simulink model "controllo_test"  (R2020a)
settings: Solver=VariableStepAuto  StartTime=0.0  StopTime=100  RelTol=1e-3
values from neighbouring files (symbols this model uses):
  a = 0.35    [data.m]    (also in geodetic2nedS.m = 6378137)
  a1 = rho * D^4 * alpha1    (= 0.000388302366464)    [data.m]
  a2 = -rho * D^3 * alpha2 * (1 - omega)    (= 0.0037030698432)    [data.m]
  AHRS_bias = [0 0 0]    [data.m]
  AHRS_sample_time = 1/50    (= 0.02)    [data.m]
  AHRS_var = ([1 1 2] * pi/180).^2    [data.m]
  alpha1 = 0.0113    [data.m]
  alpha2 = -0.0091    [data.m]
  c = son2(1)    [Sonar_id.m]    (also in data.m = 0.19)
  current = [seaCurrent; 0; 0; 0]    [data.m]
  D = 0.076    [data.m]
  dead_zone_limit = 31.5    [data.m]
  DVL_sample_t = 1/12    (= 0.0833333333333)    [data.m]
  DVL_var1 = 0.005^2    (= 2.5e-05)    [data.m]
  DVL_var2 = 0.015^2    (= 0.000225)    [data.m]
  DVL_var3 = 0.023^2    (= 0.000529)    [data.m]
  gps_sample_t = 1    [data.m]
  H = eye(3)    [data.m]    (also in navigation_data.m)
  IMU_sample_time = 1/100    (= 0.01)    [data.m]
  initial = []    [data.m]
  INSP = unicode2native(inspectionDirection)    [data.m]
  Ki_bodypos1 = 0    [parametri_PID.m]
  Ki_bodypos2 = 0    [parametri_PID.m]
  Ki_bodypos3 = 0    [parametri_PID.m]
  Ki_bodypos4 = 0    [parametri_PID.m]
  Ki_bodypos5 = 0    [parametri_PID.m]
  Ki_depth1 = 0    [parametri_PID.m]
  Ki_depth2 = 0    [parametri_PID.m]
  Ki_depth3 = 0    [parametri_PID.m]
  Ki_depth4 = 0    [parametri_PID.m]
  Ki_depth5 = 0    [parametri_PID.m]
  Ki_latvel1 = 0    [parametri_PID.m]
  Ki_latvel2 = 0    [parametri_PID.m]
  Ki_latvel3 = 0    [parametri_PID.m]
  Ki_latvel4 = 0    [parametri_PID.m]
  Ki_latvel5 = 0    [parametri_PID.m]
  Ki_P1 = 0    [parametri_PID.m]
  Ki_P2 = 0    [parametri_PID.m]
  Ki_P3 = 0    [parametri_PID.m]
  Ki_P4 = 0    [parametri_PID.m]
  Ki_P5 = 0    [parametri_PID.m]
  Ki_R1 = 0    [parametri_PID.m]
  Ki_R2 = 0    [parametri_PID.m]
  Ki_R3 = 0    [parametri_PID.m]
  Ki_R4 = 0    [parametri_PID.m]
  Ki_R5 = 0    [parametri_PID.m]
  Ki_rel_or1 = 0    [parametri_PID.m]
  Ki_rel_or2 = 0    [parametri_PID.m]
  Ki_rel_or3 = 0    [parametri_PID.m]
  Ki_rel_or4 = 0    [parametri_PID.m]
  Ki_rel_or5 = 0    [parametri_PID.m]
  Ki_reldist1 = 0    [parametri_PID.m]
  Ki_reldist2 = 0    [parametri_PID.m]
  Ki_reldist3 = 0    [parametri_PID.m]
  Ki_reldist4 = 0    [parametri_PID.m]
  Ki_reldist5 = 0    [parametri_PID.m]
  Ki_surge1 = 0    [parametri_PID.m]
  Ki_surge2 = 0    [parametri_PID.m]
  Ki_surge3 = 0    [parametri_PID.m]
  Ki_surge4 = 0    [parametri_PID.m]
  Ki_surge5 = 0    [parametri_PID.m]
  Ki_yaw1 = 0    [parametri_PID.m]
  Ki_yaw2 = 0    [parametri_PID.m]
  Ki_yaw3 = 0    [parametri_PID.m]
  Ki_yaw4 = 0    [parametri_PID.m]
  Ki_yaw5 = 0    [parametri_PID.m]
  Kp_bodypos1 = 0    [parametri_PID.m]
  Kp_bodypos2 = 2    [parametri_PID.m]
  Kp_bodypos3 = 2    [parametri_PID.m]
  Kp_bodypos4 = 2    [parametri_PID.m]
  Kp_bodypos5 = 2    [parametri_PID.m]
  Kp_depth1 = 0    [parametri_PID.m]
  Kp_depth2 = 2    [parametri_PID.m]
  Kp_depth3 = 2    [parametri_PID.m]
  Kp_depth4 = 2    [parametri_PID.m]
  Kp_depth5 = 2    [parametri_PID.m]
  Kp_latvel1 = 0    [parametri_PID.m]
  Kp_latvel2 = 2    [parametri_PID.m]
  Kp_latvel3 = 2    [parametri_PID.m]
  Kp_latvel4 = 2    [parametri_PID.m]
  Kp_latvel5 = 2    [parametri_PID.m]
  Kp_P1 = 0    [parametri_PID.m]
  Kp_P2 = 2    [parametri_PID.m]
  Kp_P3 = 2    [parametri_PID.m]
  Kp_P4 = 2    [parametri_PID.m]
  Kp_P5 = 2    [parametri_PID.m]
  Kp_R1 = 0    [parametri_PID.m]
  Kp_R2 = 2    [parametri_PID.m]
  Kp_R3 = 2    [parametri_PID.m]
  Kp_R4 = 2    [parametri_PID.m]
  Kp_R5 = 2    [parametri_PID.m]
  Kp_rel_or1 = 0    [parametri_PID.m]
  Kp_rel_or2 = 2    [parametri_PID.m]
  Kp_rel_or3 = 2    [parametri_PID.m]
  Kp_rel_or4 = 2    [parametri_PID.m]
  Kp_rel_or5 = 2    [parametri_PID.m]
  Kp_reldist1 = 0    [parametri_PID.m]
  Kp_reldist2 = 2    [parametri_PID.m]
  Kp_reldist3 = 2    [parametri_PID.m]
  Kp_reldist4 = 2    [parametri_PID.m]
  Kp_reldist5 = 2    [parametri_PID.m]
  Kp_surge1 = 0    [parametri_PID.m]
  Kp_surge2 = 2    [parametri_PID.m]
  Kp_surge3 = 2    [parametri_PID.m]
  Kp_surge4 = 2    [parametri_PID.m]
  Kp_surge5 = 2    [parametri_PID.m]
  Kp_yaw1 = 0.6*6    (= 3.6)    [parametri_PID.m]
  Kp_yaw2 = 2    [parametri_PID.m]
  Kp_yaw3 = 2    [parametri_PID.m]
  Kp_yaw4 = 2    [parametri_PID.m]
  Kp_yaw5 = 2    [parametri_PID.m]
  M = M_rb + M_a    [Masse.m]
  M_inv = inv(M)    [Masse.m]
  n_max = 340    [data.m]
  num_cycle = 5    [data.m]    (also in navigation_data.m)
  omega = 0.1    [data.m]
  ps_sample_t = 0.02    [data.m]
  ps_var = (5000/3)^2    (= 2777777.77778)    [data.m]
  pylonCenter = [ 43.723046 ... (first row only)    [missionB.m]
  pylonRadius = 10    [missionB.m]
  ... (+3 more)
undefined symbols (not defined in the file or in its folder): arrival_point, DiscIntNeverNeededParam, Kd_bodypos2, Kd_bodyposy2, Kd_dist_mis2, Kd_surge2, Kd_yaw1, Ki_bodyposy2, Ki_dist_mis2, Kp_dist_mis2, s_data
libraries: simulink x8
(part 1 of 4)
settings Model: Creator=andrea  LastModifiedBy=marco
settings DebuggingCC: ArithmeticOperatorsInVariantConditions=warning
settings SFSimCC: CustomCodeUndefinedFunction=UseInterfaceOnly

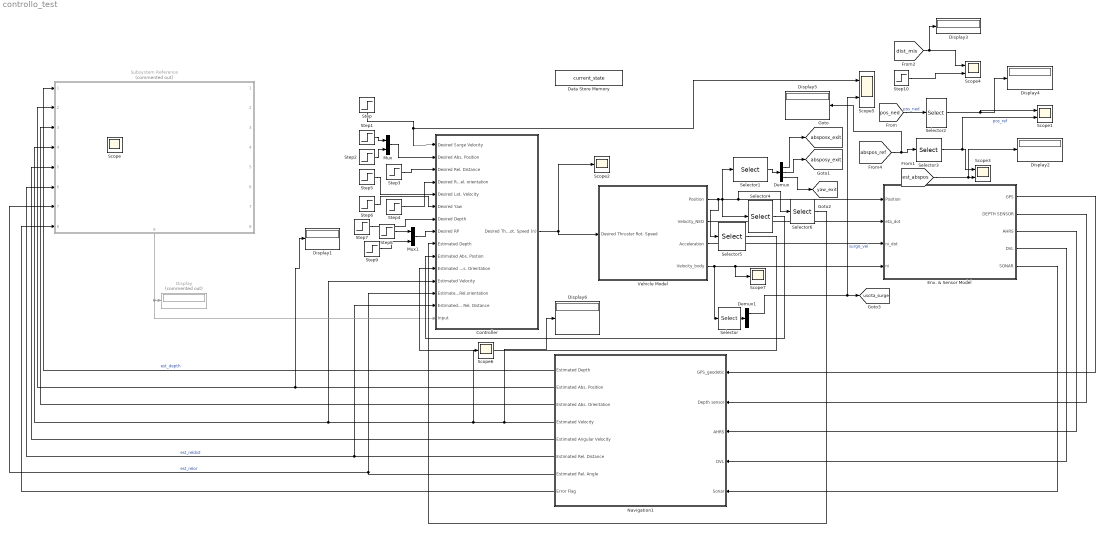
== system controllo_test ==
  Controller : Subsystem
  Data Store Memory : DataStoreMemory  DataStoreName=current_state  ReadBeforeWriteMsg=warning  WriteAfterWriteMsg=warning  WriteAfterReadMsg=warning  ShowAdditionalParam=off
  Demux : Demux  Outputs=3
  Demux1 : Demux  Outputs=2
  Display : Display  Commented=on
  Display{1..6} (6 alike) : Display
  Env. & Sensor Model : Subsystem
  Mux : Mux  Inputs=2
  Mux1 : Mux  Inputs=2
  Navigation1 : Subsystem
  Scope{1,3..5} (4 alike) : Scope  NumInputPorts=2
  Scope{,2,6..7} (4 alike) : Scope
  Selector : Selector  InputPortWidth=6  IndexOptions=Index vector (dialog)  Indices=[1 2 ]  OutputSizes=1
  Selector1 : Selector  InputPortWidth=6  IndexOptions=Index vector (dialog)  Indices=[1 2 6]  OutputSizes=1
  Selector2 : Selector  InputPortWidth=6  IndexOptions=Index vector (dialog)  Indices=[1 2]  OutputSizes=1
  Selector3 : Selector  InputPortWidth=3  IndexOptions=Index vector (dialog)  Indices=[1 2]  OutputSizes=1
  Selector4 : Selector  InputPortWidth=6  IndexOptions=Index vector (dialog)  Indices=[1 2 ]  OutputSizes=1
  Selector5 : Selector  InputPortWidth=6  IndexOptions=Index vector (dialog)  Indices=[4 5 6]  OutputSizes=1
  Selector6 : Selector  InputPortWidth=6  IndexOptions=Index vector (dialog)  Indices=[3]  OutputSizes=1
  Step{,3..8,10} (8 alike) : Step  After=0  SampleTime=0
  Step1 : Step  After=43.722904747658461  SampleTime=0
  Step2 : Step  After=10.396596368122747  SampleTime=0
  Step9 : Step  SampleTime=0
  Subsystem Reference : Subsystem  Commented=on  ReferencedSubsystem=mission_supervisor_sys
      settings: PortSchema="{\"entries\":[{\"content\":{\"sides\":[{\"content\":{\"connectorIds\":[\"In1\",\"In2\",\"In3\",\"In4\",\"In5\",\"In6\",\"In7\",\"In8\"]},\"type\":\"ConnectorPlacement.EquallySpacedRectSide\",\"uuid\":\"88d2dc79-848e-42f0-9e9e-23d8acdf1ba5\"},{\"content\":{\"connectorIds\":[\"Out1\",\"Out2\",\"Out3\",\"Out4\",\"Out5\",\"Out6\",\"Out7\",\"Out8\"],\"side\":\"RIGHT\"},\"type\":\"ConnectorPlacement.EquallySpacedRectSide\",\"uuid\":\"9b84f7d8-cdab-4722-ae5c-2c9e65c7a82f\"},{\"content\":{\"connectorIds\":[],\"side\":\"TOP\"},\"type\":\"ConnectorPlacement.EquallySpacedRectSide\",\"uuid\":\"41854cae-679a-477c-a337-a695a7e6b935\"},{\"content\":{\"connectorIds\":[\"Out9\"],\"side\":\"BOTTOM\"},\"type\":\"ConnectorPlacement.EquallySpacedRectSide\",\"uuid\":\"9cd3ab99-0ab4-4818-acd3-672b60d7f95d\"}]},\"type\":\"ConnectorPlacement.EquallySpacedConnector\",\"uuid\":\"a3d82e32-8d54-4351-960a-48f312f72e96\"}],\"packageUris\":[\"http://schema.mathworks.com/mf0/Connector/19700101\"],\"version\":\"1.0\"}"
  Vehicle Model : Subsystem
      mask Display: image('$imagefile'); % Use "Edit Image" on toolstrip to change.
  tag scope: absposx_exit=global, absposy_exit=global, uscita_surge=global, yaw_exit=global
  wires:
  Controller/1(Desired Thruster Rot. Speed (n)) -> Vehicle Model/1(Desired Thruster Rot. Speed), Scope2/1
  Vehicle Model/1(Position) -> Selector5/1, Selector4/1, Selector1/1, Selector6/1, Env. & Sensor Model/1(Position)
  Env. & Sensor Model/2(DEPTH SENSOR) -> Navigation1/2(Depth sensor)
  Env. & Sensor Model/3(AHRS) -> Navigation1/3(AHRS)
  Navigation1/1(Estimated Depth) -> Subsystem Reference/1  "est_depth"
  Navigation1/3(Estimated Abs. Orientation) -> Subsystem Reference/3
  Navigation1/4(Estimated Velocity) -> Display6/1, Scope6/1, Subsystem Reference/4, Controller/12(Estimated Velocity)
  Vehicle Model/4(Velocity_body) -> Scope7/1, Env. & Sensor Model/4(ni), Selector/1
  Navigation1/6(Estimated Rel. Distance) -> Subsystem Reference/6, Controller/14(Estimated Rel. Distance)  "est_reldist"
  Navigation1/7(Estimated Rel. Angle) -> Subsystem Reference/7, Controller/13(Estimated Rel.orientation)  "est_relor"
  Vehicle Model/2(Velocity_NED) -> Env. & Sensor Model/2(eta_dot)
  Vehicle Model/3(Acceleration) -> Env. & Sensor Model/3(ni_dot)
  Env. & Sensor Model/1(GPS) -> Navigation1/1(GPS_geodetic)
  Env. & Sensor Model/4("DVL ") -> Navigation1/4(DVL)
  Env. & Sensor Model/5(SONAR) -> Navigation1/5(Sonar)
  Subsystem Reference/9 -> Controller/15(Input), Display/1
  Navigation1/5(Estimated Angular Velocity) -> Subsystem Reference/5
  Navigation1/8(Error Flag) -> Subsystem Reference/8
  Step/1 -> Scope5/1, Controller/1(Desired Surge Velocity)
  Step2/1 -> Mux/2
  Mux/1 -> Controller/2(Desired Abs. Position)
  Selector/1 -> Demux1/1
  Demux1/1 -> Scope5/2, [uscita_surge]  "surge_vel"
  Step3/1 -> Controller/3(Desired Rel. Distance)
  Step4/1 -> Controller/4(Desired Rel. orientation)
  Step5/1 -> Controller/5(Desired Lat. Velocity)
  Step6/1 -> Controller/6(Desired Yaw)
  Step7/1 -> Controller/7(Desired Depth)
  Step9/1 -> Mux1/2
  Step8/1 -> Mux1/1
  Mux1/1 -> Controller/8(Desired RP)
  Step1/1 -> Mux/1
  [abspos_ref] -> Display5/1, Selector3/1
  [pos_ned] -> Selector2/1  "pos_ned"
  Selector3/1 -> Scope1/2, Scope3/1  "pos_ref"
  Selector1/1 -> Demux/1
  Demux/3 -> [yaw_exit]
  Demux/1 -> [absposx_exit]
  Demux/2 -> [absposy_exit]
  [est_abspos] -> Display2/1, Scope3/2
  [dist_mis] -> Display3/1, Scope4/1
  Step10/1 -> Scope4/2
  Selector2/1 -> Scope1/1, Display4/1
  Navigation1/2(Estimated Abs. Position) -> Subsystem Reference/2, Display1/1
  Selector4/1 -> Controller/10(Estimated Abs. Postion)
  Selector5/1 -> Controller/11(Estimated Abs. Orientation)
  Selector6/1 -> Controller/9(Estimated Depth)

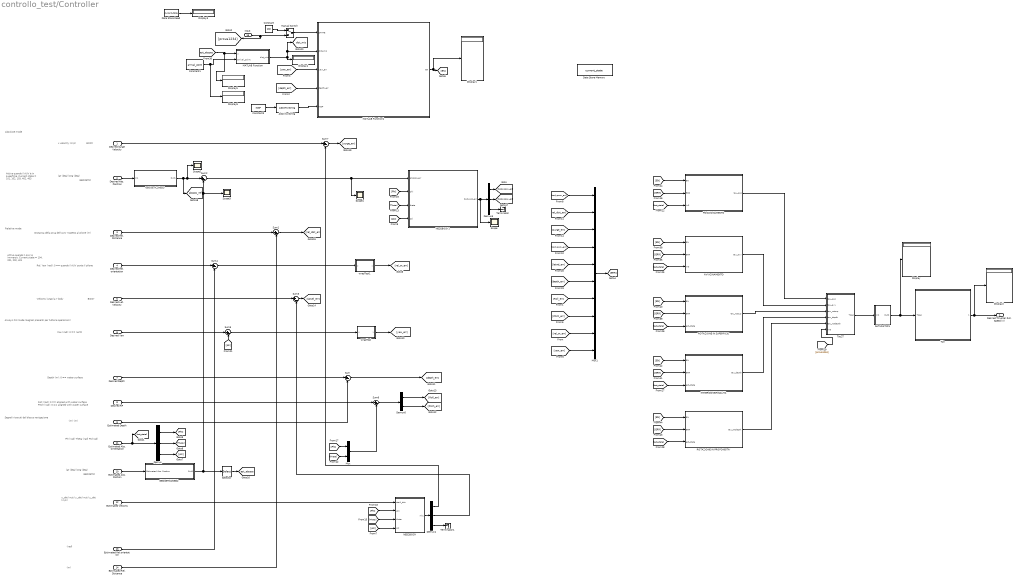
== system controllo_test/Controller ==
  note: lat (deg)
      | long (deg)
  note: (m)
  note: BODY
  note: x velocity (m/s)
  note: lat (deg)
      | long (deg)
  note: GEODETIC
  note: BODY
  note: Relative mode
  note: Absolute mode
  note: GEODETIC
  note: Always ON mode (segnali presenti per tutte le operazioni)
  note: Roll (rad): 0 == aligned with water surface
      | Pitch (rad): 0 == aligned with water surface
  note: Velocity lungo la Y body
  note: Distanza della prua dell'AUV rispetto al pilone (m)
  note: Rel. Yaw (rad): 0 == quando il AUV punta il pilone
  note: Attiva quando il AUV è immerso.
      | Current state = 104, 201, 202, 401
  note: Attiva quando il AUV è in superficie.
      | Current state = 101, 102, 103, 402, 403
  note: Depth (m): 0 == water surface
  note: x_dot        (m/s)
      | y_dot          (m/s)
      | z_dot         (m/s)
  note: (rad)
  note: Segnali ricevuti dal blocco navigazione
  note: (m)
      | (m)
  note: Yaw (rad): 0 == north
  note: Phi (rad)
      | Theta (rad)
      | Psi(rad)
  Desired Surge Velocity : Inport
  Desired Abs. Position : Inport  Port=2  Unit=deg  PortDimensions=2
  Desired Rel. Distance : Inport  Port=3  Unit=m  PortDimensions=1
  Desired Rel. orientation : Inport  Port=4  Unit=rad  PortDimensions=1
  Desired Lat. Velocity : Inport  Port=5  Unit=m/s  PortDimensions=1
  Desired Yaw : Inport  Port=6  Unit=rad  PortDimensions=1
  Desired Depth : Inport  Port=7  Unit=m  PortDimensions=1
  Desired RP : Inport  Port=8  Unit=rad  PortDimensions=2
  Estimated Depth : Inport  Port=9  Unit=m  PortDimensions=1
  Estimated Abs. Postion : Inport  Port=10  Unit=deg  PortDimensions=2
  Estimated Abs. Orientation : Inport  Port=11  Unit=rad  PortDimensions=3
  Estimated Velocity : Inport  Port=12  Unit=m/s  PortDimensions=3
  Estimated Rel.orientation : Inport  Port=13  Unit=rad  PortDimensions=1
  Estimated Rel. Distance : Inport  Port=14  Unit=m  PortDimensions=1
  Input : Inport  Port=15
  ASCII to String : ASCIIToString
  AVVICINAMENTO : Subsystem
  Constant : Constant  Value=102
  Constant1 : Constant  Value=arrival_point
  Constant3 : Constant  Value=INSP  OutDataTypeStr=uint8
  Data Store Memory : DataStoreMemory  DataStoreName=current_state  ReadBeforeWriteMsg=warning  WriteAfterWriteMsg=warning  WriteAfterReadMsg=warning  ShowAdditionalParam=off
  Data Store Read : DataStoreRead  DataStoreName=current_state  SampleTime=0.1
  Demux : Demux  Outputs=3
  Demux1 : Demux  Outputs=3
  Demux5 : Demux  Outputs=3
  Demux6 : Demux  Outputs=2
  Display{,1..6} (7 alike) : Display
  GEODETIC2NED2 : Subsystem
  GEODETIC2NED3 : Subsystem
  IMMERSIONE/RISALITA : Subsystem
  MATLAB Function : MATLAB Function  TreatAsAtomicUnit=on
  MATLAB Function1 : MATLAB Function  TreatAsAtomicUnit=on  SystemSampleTime=0.1
  Manual Switch : ManualSwitch
  Mux : Mux  Inputs=2
  Mux1 : Mux  Inputs=10
  NED2BODY : MATLAB Function  TreatAsAtomicUnit=on
  NED2BODY1 : MATLAB Function  TreatAsAtomicUnit=on
  POSIZIONAMENTO : Subsystem
  ROTAZIONE IN PROFONDITA' : Subsystem
  ROTAZIONE IN SUPERFICIE : Subsystem
  SATURATION : Subsystem
  Scope{,1..3} (4 alike) : Scope
  Selector : Selector  InputPortWidth=3  IndexOptions=Index vector (dialog)  Indices=[1 2]  OutputSizes=1
  Sum{,1..7} (8 alike) : Sum  Inputs=|+-
  T2n : Subsystem
  Tau2T : Subsystem
  Terminator : Terminator
  Terminator1 : Terminator
  wrapTopi : MATLAB Function  TreatAsAtomicUnit=on
  wrapTopi1 : MATLAB Function  TreatAsAtomicUnit=on
  Desired Thruster Rot. Speed (n) : Outport  Unit=rad/s  PortDimensions=7
  tag scope: abspos_ref=global, dist_mis=global, est_abspos=global
  wires:
  Estimated Abs. Orientation/1 -> [est_state], Demux/1
  Desired Depth/1 -> Sum/1
  Estimated Depth/1 -> Sum/2
  Mux/1 -> Sum6/2
  Desired RP/1 -> Sum6/1
  T2n/1(n) -> Display2/1, Desired Thruster Rot. Speed (n)/1
  Desired Lat. Velocity/1 -> Sum3/1
  Desired Rel. Distance/1 -> Sum1/1
  Estimated Rel. Distance/1 -> Sum1/2
  Sum2/1 -> Scope1/1, NED2BODY1/1(abspos_err)
  Desired Abs. Position/1 -> GEODETIC2NED3/1(In1)
  GEODETIC2NED3/1(Out1) -> [abspos_ref], Sum2/1, Scope2/1
  Estimated Abs. Postion/1 -> GEODETIC2NED2/1(Estimated Abs. Postion)
  GEODETIC2NED2/1(Out1) -> Selector/1, Scope3/1, Sum2/2
  Demux1/1 -> Sum7/2
  Demux1/2 -> Sum3/2
  NED2BODY/1(mi1) -> Demux1/1
  Estimated Velocity/1 -> NED2BODY/1(eta1_dot)
  Estimated Rel.orientation/1 -> Sum4/2
  Demux/3 -> [psi]
  [psi] -> NED2BODY/4(psi)
  [psi] -> NED2BODY1/4(psi)
  Demux/2 -> [Theta]
  [Theta] -> Mux/2
  [Theta] -> NED2BODY1/3(theta)
  [Theta] -> NED2BODY/3(theta)
  Demux/1 -> [Phi]
  [Phi] -> Mux/1
  [Phi] -> NED2BODY/2(phi)
  [Phi] -> NED2BODY1/2(phi)
  Tau2T/1(Tdes) -> SATURATION/1(In2)
  SATURATION/1(Out2) -> Display/1, T2n/1(Tdes)
  Desired Rel. orientation/1 -> Sum4/1
  Desired Surge Velocity/1 -> Sum7/1
  [ERR] -> POSIZIONAMENTO/2(ERR)
  [EN] -> POSIZIONAMENTO/1(EN)
  Sum4/1 -> wrapTopi1/1(u)
  Desired Yaw/1 -> Sum5/1
  [psi] -> Sum5/2
  Sum/1 -> [depth_err]
  Sum3/1 -> [latvel_err]
  Sum1/1 -> [rel_dist_err]
  NED2BODY1/1(bodypos_err) -> Scope/1, Demux5/1
  Sum7/1 -> [surge_err]
  Demux5/1 -> [bodyposx_err]
  Demux5/2 -> [bodyposy_err]
  [EN] -> AVVICINAMENTO/1(EN)
  [ERR] -> AVVICINAMENTO/2(ERR)
  [ERR] -> ROTAZIONE IN SUPERFICIE/2(ERR)
  [ERR] -> IMMERSIONE/RISALITA/2(ERR)
  [EN] -> IMMERSIONE/RISALITA/1(EN)
  [ERR] -> ROTAZIONE IN PROFONDITA'/2(ERR)
  [EN] -> ROTAZIONE IN PROFONDITA'/1(EN)
  MATLAB Function1/1(EN) -> [EN], Display1/1
  [bodyposx_err] -> Mux1/1
  [rel_dist_err] -> Mux1/2
  [surge_err] -> Mux1/3
  [bodyposy_err] -> Mux1/4
  [latvel_err] -> Mux1/5
  [depth_err] -> Mux1/6
  Mux1/1 -> [ERR]
  [Roll_err] -> Mux1/7
  [Pitch_err] -> Mux1/8
  [rel_or_err] -> Mux1/9
  [yaw_err] -> Mux1/10
  [EN] -> ROTAZIONE IN SUPERFICIE/1(EN)
  POSIZIONAMENTO/1(tau_pos) -> Tau2T/1(tau_pos)
  AVVICINAMENTO/1(tau_avv) -> Tau2T/2(tau_avv)
  ROTAZIONE IN SUPERFICIE/1(tau_rotsup) -> Tau2T/3(tau_rotsup)
  IMMERSIONE/RISALITA/1(tau_depth) -> Tau2T/4(tau_depth)
  ROTAZIONE IN PROFONDITA'/1(tau_rotdepth) -> Tau2T/5(tau_rotdepth)
  [depth_err] -> MATLAB Function1/4(depth_err)
  [yaw_err] -> MATLAB Function1/3(yaw_err)
  Constant/1 -> Manual Switch/1
  Data Store Read/1 -> Display3/1
  Manual Switch/1 -> MATLAB Function1/1(STATE)
  Demux5/3 -> Terminator/1
  wrapTopi1/1(y) -> [rel_or_err]
  wrapTopi/1(y) -> [yaw_err]
  Sum6/1 -> Demux6/1
  Demux6/1 -> [Roll_err]
  Demux6/2 -> [Pitch_err]
  ASCII to String/1 -> MATLAB Function1/5(INSP)
  Constant3/1 -> ASCII to String/1
  [est_state] -> POSIZIONAMENTO/3(In3)
  [est_state] -> AVVICINAMENTO/3(In3)
  [est_state] -> ROTAZIONE IN SUPERFICIE/3(est_state)
  [est_state] -> IMMERSIONE/RISALITA/3(est_state)
  [est_state] -> ROTAZIONE IN PROFONDITA'/3(est_state)
  Demux1/3 -> Terminator1/1
  Input/1 -> Manual Switch/2, [prova1234]
  [prova1234] -> Tau2T/6(In6)
  Sum5/1 -> wrapTopi/1(u)
  Selector/1 -> [est_abspos]
  [est_abspos] -> Display5/1, MATLAB Function/1(u)
  Constant1/1 -> Display6/1, MATLAB Function/2(arrival_point)
  MATLAB Function/1(dist_mis) -> [dist_mis], MATLAB Function1/2(dist_mis), Display4/1

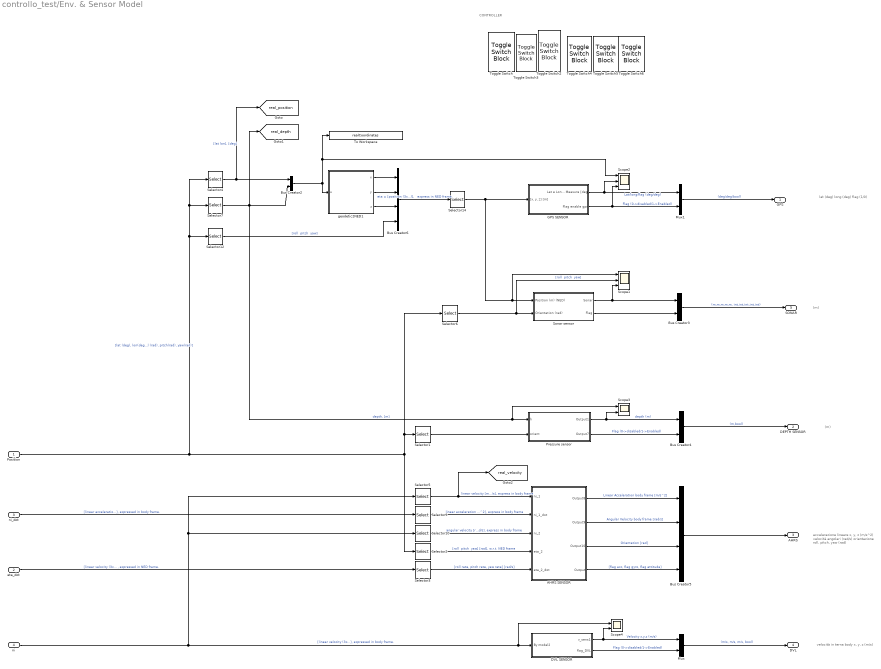
== system controllo_test/Env. & Sensor Model ==
  note: (m)
  note: velocità in terna body x, y, z (m/s)
  note: accelerazione lineare x, y, z (m/s^2)
      | velocità angolari (rad/s)
      | orientazione roll, pitch, yaw (rad)
  note: (m)
  note: lat (deg)
      | long (deg)
      | flag (1/0)
  note: CONTROLLER
  Position : Inport
  eta_dot : Inport  Port=2
  ni_dot : Inport  Port=3
  ni : Inport  Port=4
  AHRS SENSOR : Subsystem
  Bus Creator2 : BusCreator  Inputs=2
  Bus Creator3 : BusCreator  Inputs=2
  Bus Creator4 : BusCreator  Inputs=2
  Bus Creator5 : BusCreator  Inputs=4
  Bus Creator6 : BusCreator  Inputs=4
  DVL SENSOR : Subsystem
  GPS SENSOR : Subsystem
  Mux : Mux  Inputs=2
  Mux1 : Mux  Inputs=2
  Pressure sensor : Subsystem
  Scope1 : Scope  NumInputPorts=3
  Scope2 : Scope  NumInputPorts=3
  Scope3 : Scope  NumInputPorts=2
  Scope4 : Scope  NumInputPorts=2
  Selector{1..3,6,10,12} (6 alike) : Selector  InputPortWidth=6  IndexOptions=Index vector (dialog)  Indices=[4 5 6]  OutputSizes=1
  Selector14 : Selector  InputPortWidth=6  IndexOptions=Index vector (dialog)  Indices=[1 2 3]  OutputSizes=1
  Selector4 : Selector  InputPortWidth=6  IndexOptions=Index vector (dialog)  Indices=[1 2]  OutputSizes=1
  Selector5 : Selector  InputPortWidth=6  IndexOptions=Index vector (dialog)  Indices=[1 2 3]  OutputSizes=1
  Selector7 : Selector  InputPortWidth=6  IndexOptions=Index vector (dialog)  Indices=[3]  OutputSizes=1
  Selector9 : Selector  InputPortWidth=6  IndexOptions=Index vector (dialog)  Indices=[1 2 3]  OutputSizes=1
  Sonar sensor : Subsystem
  To Workspace : ToWorkspace  VariableName=realCoordinates  SampleTime=-1
  Toggle Switch{,2..6} (6 alike) : ToggleSwitchBlock
  geodetic2NED1 : MATLAB Function  TreatAsAtomicUnit=on
  GPS : Outport
  DEPTH SENSOR : Outport  Port=2
  AHRS : Outport  Port=3
  "DVL " : Outport  Port=4
  SONAR : Outport  Port=5
  tag scope: real_depth=global, real_position=global, real_velocity=global
  wires:
  Pressure sensor/1(Output1) -> Bus Creator4/1, Scope3/2  "depth (m)"
  AHRS SENSOR/1(Output8) -> Bus Creator5/1  "Linear Acceleration body frame [m/s^2]"
  Mux1/1 -> GPS/1  "(deg/deg/bool)"
  AHRS SENSOR/3(Output10) -> Bus Creator5/3  "Orientation [rad]"
  Bus Creator6/1 -> Selector14/1  "eta = [position (3x1),  \t  orientation (3x1)], \t  express in NED frame."
  Selector14/1 -> GPS SENSOR/1("[x, y, z] [m]"), Sonar sensor/1(Position (m) (NED)), Scope1/1
  GPS SENSOR/1(Lat e Lon Measure [deg]) -> Scope2/2, Mux1/1  "Lat/long/flag (deg/deg)"
  Selector7/1 -> Bus Creator2/2, [real_depth], Scope3/1, Pressure sensor/1(h)  "depth, [m]"
  geodetic2NED1/3(z) -> Bus Creator6/3
  Selector2/1 -> AHRS SENSOR/4(eta_2)  "[roll  pitch  yaw] [rad], w.r.t. NED frame"
  Bus Creator5/1 -> AHRS/1
  AHRS SENSOR/2(Output9) -> Bus Creator5/2  "Angular Velocity body frame [rad/s]"
  ni/1 -> DVL SENSOR/1(By model2), Scope4/1, Selector10/1, Selector5/1  "[linear velocity (3x1),angular velocity (3x1)], expressed in body frame."
  Selector6/1 -> Sonar sensor/2(Orientation (rad)), Scope1/2  "[roll  pitch  yaw]"
  AHRS SENSOR/4(Output) -> Bus Creator5/4  "[flag acc, flag gyro, flag attitude]"
  GPS SENSOR/2(Flag enable gps) -> Scope2/3, Mux1/2  "Flag (0->disabled/1->Enabled)"
  Selector10/1 -> AHRS SENSOR/3(ni_2)  "angular velocity [rad/s], express in body frame"
  eta_dot/1 -> Selector3/1  "[linear velocity (3x1), roll rate, pitch rate, yaw rate] , expressed in NED frame."
  Selector9/1 -> AHRS SENSOR/2(ni_1_dot)  "linear acceleration [m/s^2], express in body frame"
  Pressure sensor/2(Output7) -> Bus Creator4/2  "Flag (0->disabled/1->Enabled)"
  Selector4/1 -> [real_position], Bus Creator2/1  "[lat lon], [deg]"
  DVL SENSOR/2(flag_DVL) -> Mux/2  "Flag (0->disabled/1->Enabled)"
  Mux/1 -> "DVL "/1  "(m/s, m/s, m/s, bool)"
  geodetic2NED1/1(x) -> Bus Creator6/1
  geodetic2NED1/2(y) -> Bus Creator6/2
  Selector3/1 -> AHRS SENSOR/5(eta_2_dot)  "[roll rate, pitch rate, yaw rate] [rad/s]"
  Sonar sensor/1(Sonar) -> Scope1/3, Bus Creator3/1
  Position/1 -> Selector2/1, Selector1/1, Selector6/1, Selector4/1, Selector7/1, Selector12/1  "[lat (deg), lon(deg), depth(m), roll (rad), pitch(rad), yaw(rad)]"
  Bus Creator4/1 -> DEPTH SENSOR/1  "(m,bool)"
  Selector5/1 -> [real_velocity], AHRS SENSOR/1(ni_1)  "linear velocity [m/s], express in body frame"
  ni_dot/1 -> Selector9/1  "[linear acceleration (3x1), angular acceleration (3x1)], expressed in body frame."
  Bus Creator2/1 -> To Workspace/1, Scope2/1, geodetic2NED1/1(u)
  DVL SENSOR/1(v_sens1) -> Scope4/2, Mux/1  "Velocity x,y,z (m/s)"
  Bus Creator3/1 -> SONAR/1  "(m,m,m,m,m, int,int,int,int,int)"
  Sonar sensor/2(Flag) -> Bus Creator3/2
  Selector12/1 -> Bus Creator6/4  "[roll  pitch  yaw]"
  Selector1/1 -> Pressure sensor/2(orient)

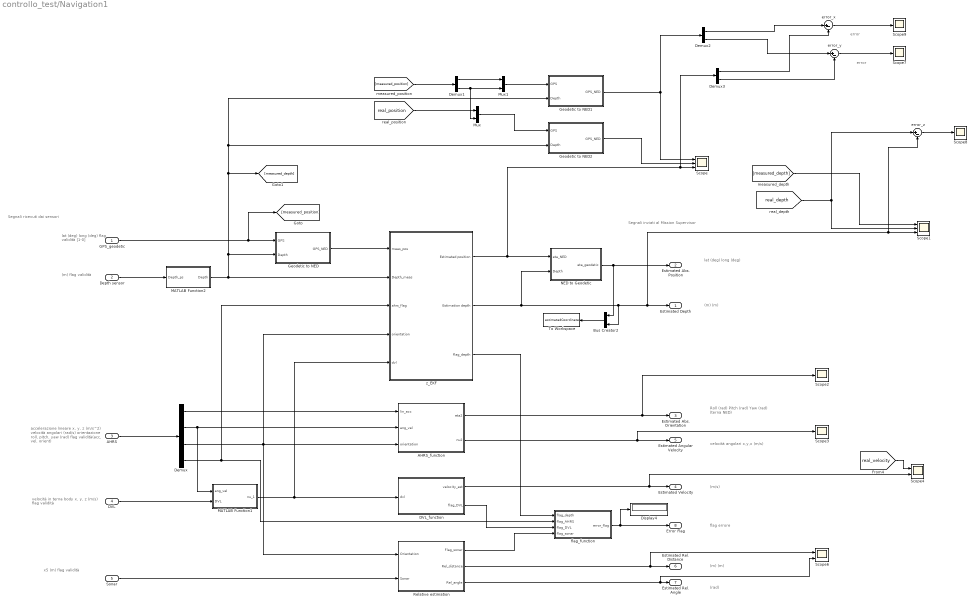
== system controllo_test/Navigation1 ==
  note: (m/s)
  note: (rad)
  note: (m)
      | (m)
  note: (m)
      | flag validità
  note: velocità in terna body x, y, z (m/s)
      | flag validità
  note: error
  note: Segnali ricevuti dai sensori
  note: flag errore
  note: accelerazione lineare x, y, z (m/s^2)
      | velocità angolari (rad/s)
      | orientazione roll, pitch, yaw (rad)
      | flag validità(acc, vel, orient)
  note: velocità angolari x,y,x (m/s)
  note: lat     (deg)
      |  long  (deg)
  note: (m)
      | (m)
  note: Roll (rad)
      | Pitch (rad)
      | Yaw (rad)
      | (terna NED)
  note: x5
      | (m)
      | flag validità
  note: Segnali inviati al Mission Supervisor
  note: error
  note: lat     (deg)
      |  long  (deg)
      | flag validità [1-0]
  GPS_geodetic : Inport  PortDimensions=3
  Depth sensor : Inport  Port=2  PortDimensions=2
  AHRS : Inport  Port=3  PortDimensions=12
  DVL : Inport  Port=4  PortDimensions=4
  Sonar : Inport  Port=5
  AHRS_function : MATLAB Function  TreatAsAtomicUnit=on
  Bus Creator2 : BusCreator  Inputs=2
  DVL_function : MATLAB Function  TreatAsAtomicUnit=on
  Demux : Demux  Outputs=[3 3 3 3]
  Demux1 : Demux  Outputs=2
  Demux2 : Demux  Outputs=2
  Demux3 : Demux  Outputs=2
  Display4 : Display
  Geodetic to NED : Subsystem
  Geodetic to NED1 : Subsystem
  Geodetic to NED2 : Subsystem
  MATLAB Function1 : MATLAB Function  TreatAsAtomicUnit=on  SystemSampleTime=DVL_sample_t
  MATLAB Function2 : MATLAB Function  TreatAsAtomicUnit=on
  Mux : Mux  Inputs=2
  Mux1 : Mux  Inputs=2
  NED to Geodetic : Subsystem
  Relative estimation : Subsystem
  Scope : Scope  NumInputPorts=3
  Scope1 : Scope  NumInputPorts=3
  Scope{2..3,7..9} (5 alike) : Scope
  Scope4 : Scope  NumInputPorts=2
  Scope6 : Scope  NumInputPorts=2
  To Workspace : ToWorkspace  VariableName=estimatedCoordinates  SampleTime=-1
  error_x : Sum  Inputs=|+-
  error_y : Sum  Inputs=|+-
  error_z : Sum  Inputs=|+-
  flag_function : MATLAB Function  TreatAsAtomicUnit=on  SystemSampleTime=1/200
  z_EKF : Subsystem
  Estimated Depth : Outport
  Estimated Abs. Position : Outport  Port=2
  Estimated Abs. Orientation : Outport  Port=3
  Estimated Velocity : Outport  Port=4
  Estimated Angular Velocity : Outport  Port=5
  Estimated Rel. Distance : Outport  Port=6
  Estimated Rel. Angle : Outport  Port=7
  Error Flag : Outport  Port=8
  wires:
  Demux3/1 -> error_x/2
  z_EKF/1(Estimated position) -> Demux3/1, Scope/3, NED to Geodetic/1(eta_NED)
  [real_velocity] -> Scope4/1
  Demux2/2 -> error_y/1
  Relative estimation/1(Flag_sonar) -> flag_function/4(flag_sonar)
  error_x/1 -> Scope9/1
  Mux/1 -> Geodetic to NED2/1(GPS)
  Bus Creator2/1 -> To Workspace/1
  Demux/4 -> z_EKF/3(ahrs_flag), flag_function/2(flag_AHRS)
  MATLAB Function2/1(Depth) -> Geodetic to NED1/2(Depth), Geodetic to NED2/2(Depth), [measured_depth], Geodetic to NED/2(Depth), z_EKF/2(Depth_meas)
  NED to Geodetic/1(eta_geodetic) -> Bus Creator2/1, Estimated Abs. Position/1
  Geodetic to NED1/1(GPS_NED) -> Scope/1, Demux2/1
  z_EKF/3(flag_depth) -> flag_function/1(flag_depth)
  flag_function/1(error_flag) -> Display4/1, Error Flag/1
  AHRS_function/1(eta2) -> Scope2/1, Estimated Abs. Orientation/1
  [real_depth] -> Scope1/2, error_z/1
  Demux3/2 -> error_y/2
  DVL_function/1(velocity_est) -> Scope4/2, Estimated Velocity/1
  AHRS/1 -> Demux/1
  Sonar/1 -> Relative estimation/2(Sonar)
  Demux/2 -> MATLAB Function1/1(ang_vel), AHRS_function/2(ang_vel)
  Demux2/1 -> error_x/1
  Relative estimation/2(Rel_distance) -> Scope6/1, Estimated Rel. Distance/1
  MATLAB Function1/1(nu_1) -> z_EKF/5(dvl), DVL_function/1(dvl)
  Demux1/1 -> Mux1/1
  Demux1/2 -> Mux/2, Mux1/2
  Geodetic to NED/1(GPS_NED) -> z_EKF/1(meas_pos)
  [real_position] -> Mux/1
  error_y/1 -> Scope7/1
  z_EKF/2(Estimation depth) -> NED to Geodetic/2(Depth), Bus Creator2/2, error_z/2, Scope1/3, Estimated Depth/1
  error_z/1 -> Scope8/1
  Relative estimation/3(Rel_angle) -> Scope6/2, Estimated Rel. Angle/1
  [measured_position] -> Demux1/1
  Geodetic to NED2/1(GPS_NED) -> Scope/2
  GPS_geodetic/1 -> Geodetic to NED/1(GPS), [measured_position]
  DVL_function/2(flag_DVL) -> flag_function/3(flag_DVL)
  Depth sensor/1 -> MATLAB Function2/1(Depth_ps)
  Mux1/1 -> Geodetic to NED1/1(GPS)
  DVL/1 -> MATLAB Function1/2(DVL)
  Demux/3 -> z_EKF/4(orientation), AHRS_function/3(orientation), Relative estimation/1(Orientation)
  [measured_depth] -> Scope1/1
  AHRS_function/2(nu2) -> Scope3/1, Estimated Angular Velocity/1
  Demux/1 -> AHRS_function/1(lin_acc)

== system controllo_test/Vehicle Model ==
  note: 3x1 (m/s^2),
      | 3x1 (rad/s^2)
  note: 3x1 (m/s),
      | 3x1 (rad/s)
  note: lat (deg)
      | long (deg)
      | prof. (m),
      | roll (rad),
      | pitch (rad),
      | yaw (rad)
  note: 3x1 (m/s),
      | 3x1 (rad/s)
  Desired Thruster Rot. Speed : Inport
  Add : Sum  Inputs=+-
  Constant : Constant  Value=[100; 100; 0; 0; 0; 0; 0]
  Current : Constant  Value=current
  Demux : Demux
  MATLAB Function : MATLAB Function  TreatAsAtomicUnit=on
  Manual Switch : ManualSwitch  CurrentSetting=0
  Model Vehicle : Subsystem
      mask Display: image('$imagefile'); % Use "Edit Image" on toolstrip to change.
  Scope : Scope
  Scope1 : Scope
  Step : Step  Time=5  Before=[0;0;0;0;0;0;0]  After=[100;-100;0;0;0;0;0]  SampleTime=0
  Thrusters : Subsystem
      mask Display: image('$imagefile'); % Use "Edit Image" on toolstrip to change.
  Position : Outport
  Velocity_NED : Outport  Port=2
  Acceleration : Outport  Port=3
  Velocity_body : Outport  Port=4
  wires:
  Demux/3 -> Velocity_body/1, Add/2  "ni"
  Model Vehicle/1(Out1) -> Demux/1
  Demux/1 -> Thrusters/2(eta), MATLAB Function/1(eta), Position/1, Scope/1  "eta"
  Desired Thruster Rot. Speed/1 -> Manual Switch/2
  Manual Switch/1 -> Thrusters/1(des rot)
  Current/1 -> MATLAB Function/2(current)
  Demux/2 -> Velocity_NED/1  "eta_dot"
  Demux/4 -> Acceleration/1  "ni_dot"
  MATLAB Function/1(ni_c) -> Model Vehicle/2(ni_current), Add/1
  Add/1 -> Thrusters/3(ni)
  Constant/1 -> Manual Switch/1
  Step/1 -> ?
  Thrusters/1(tau) -> Scope1/1, Model Vehicle/1(tau)

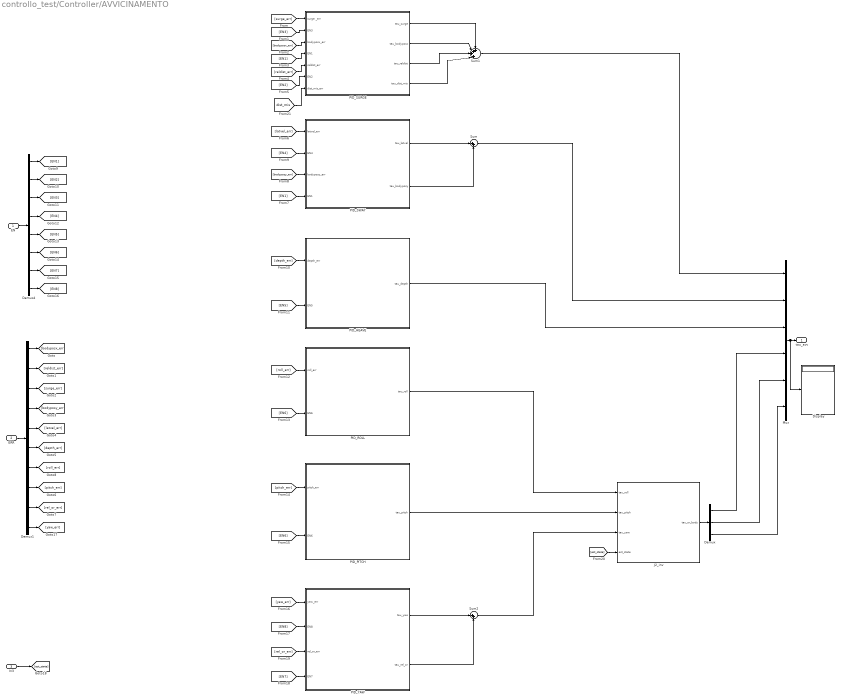
== system controllo_test/Controller/AVVICINAMENTO ==
  EN : Inport
  ERR : Inport  Port=2
  In3 : Inport  Port=3
  Demux : Demux  Outputs=3
  Demux1 : Demux  Outputs=10
  Demux4 : Demux  Outputs=8
  Display : Display
  J2_inv : MATLAB Function  TreatAsAtomicUnit=on
  Mux : Mux  Inputs=6
  PID_HEAVE : Subsystem
  PID_PITCH : Subsystem
  "PID_ROLL " : Subsystem
  PID_SURGE : Subsystem
  PID_SWAY : Subsystem
  PID_YAW : Subsystem
  Sum : Sum  Inputs=|++
  Sum1 : Sum  Inputs=++++|
  Sum2 : Sum  Inputs=|++
  tau_avv : Outport
  wires:
  EN/1 -> Demux4/1
  ERR/1 -> Demux1/1
  Demux4/1 -> [EN1]
  Demux4/2 -> [EN2]
  Demux4/3 -> [EN3]
  Demux4/4 -> [EN4]
  Demux4/5 -> [EN5]
  Demux4/6 -> [EN6]
  Demux4/7 -> [EN7]
  Demux4/8 -> [EN8]
  Demux1/1 -> [bodyposx_err]
  Demux1/2 -> [reldist_err]
  Demux1/3 -> [surge_err]
  Demux1/4 -> [bodyposy_err]
  Demux1/5 -> [latvel_err]
  Demux1/6 -> [depth_err]
  Demux1/7 -> [roll_err]
  Demux1/8 -> [pitch_err]
  Demux1/9 -> [rel_or_err]
  Demux1/10 -> [yaw_err]
  [surge_err] -> PID_SURGE/1(surge _err)
  [EN3] -> PID_SURGE/2(EN3)
  [bodyposx_err] -> PID_SURGE/3(bodyposx_err)
  [EN1] -> PID_SURGE/4(EN1)
  [reldist_err] -> PID_SURGE/5(reldist_err)
  [EN2] -> PID_SURGE/6(EN2)
  [latvel_err] -> PID_SWAY/1(latvel_err)
  [bodyposy_err] -> PID_SWAY/3(bodyposy_err)
  [depth_err] -> PID_HEAVE/1(depth_err)
  [roll_err] -> "PID_ROLL "/1(roll_err)
  [pitch_err] -> PID_PITCH/1(pitch_err)
  [EN6] -> PID_PITCH/2(EN6)
  [yaw_err] -> PID_YAW/1(yaw_err)
  [EN4] -> PID_SWAY/2(EN4)
  [EN1] -> PID_SWAY/4(EN1)
  [EN5] -> PID_HEAVE/2(EN5)
  [EN6] -> "PID_ROLL "/2(EN6)
  [EN8] -> PID_YAW/2("EN8 ")
  [EN7] -> PID_YAW/4(EN7)
  [rel_or_err] -> PID_YAW/3(rel_or_err)
  PID_HEAVE/1(tau_depth) -> Mux/3
  PID_SURGE/1(tau_surge) -> Sum1/1
  Mux/1 -> Display/1, tau_avv/1
  Sum1/1 -> Mux/1
  Sum/1 -> Mux/2
  PID_YAW/1(tau_yaw) -> Sum2/1
  PID_SWAY/2(tau_bodyposy) -> Sum/2
  PID_SURGE/3(tau_reldist) -> Sum1/3
  PID_SURGE/2(tau_bodyposx) -> Sum1/2
  PID_YAW/2(tau_rel_or) -> Sum2/2
  PID_SWAY/1(tau_latvel) -> Sum/1
  Demux/2 -> Mux/5
  PID_PITCH/1(tau_pitch) -> J2_inv/2(tau_pitch)
  J2_inv/1(tau_or_body) -> Demux/1
  Demux/3 -> Mux/6
  "PID_ROLL "/1(tau_roll) -> J2_inv/1(tau_roll)
  Demux/1 -> Mux/4
  [est_state] -> J2_inv/4(est_state)
  Sum2/1 -> J2_inv/3(tau_yaw)
  In3/1 -> [est_state]
  [dist_mis] -> PID_SURGE/7(dist_mis_err)
  PID_SURGE/4(tau_dist_mis) -> Sum1/4

== system controllo_test/Controller/GEODETIC2NED2 ==
  Estimated Abs. Postion : Inport  Unit=deg  PortDimensions=2
  GEODETIC2NED1 : Subsystem
  Out1 : Outport
  wires:
  GEODETIC2NED1/1(Out1) -> Out1/1
  Estimated Abs. Postion/1 -> GEODETIC2NED1/1(In1)

== system controllo_test/Controller/GEODETIC2NED3 ==
  In1 : Inport
  Demux2 : Demux  Outputs=2
  GEODETIC2NED : Subsystem
  Out1 : Outport
  wires:
  Demux2/2 -> GEODETIC2NED/2(lon)
  GEODETIC2NED/1(Out1) -> Out1/1
  Demux2/1 -> GEODETIC2NED/1(lat)
  In1/1 -> Demux2/1

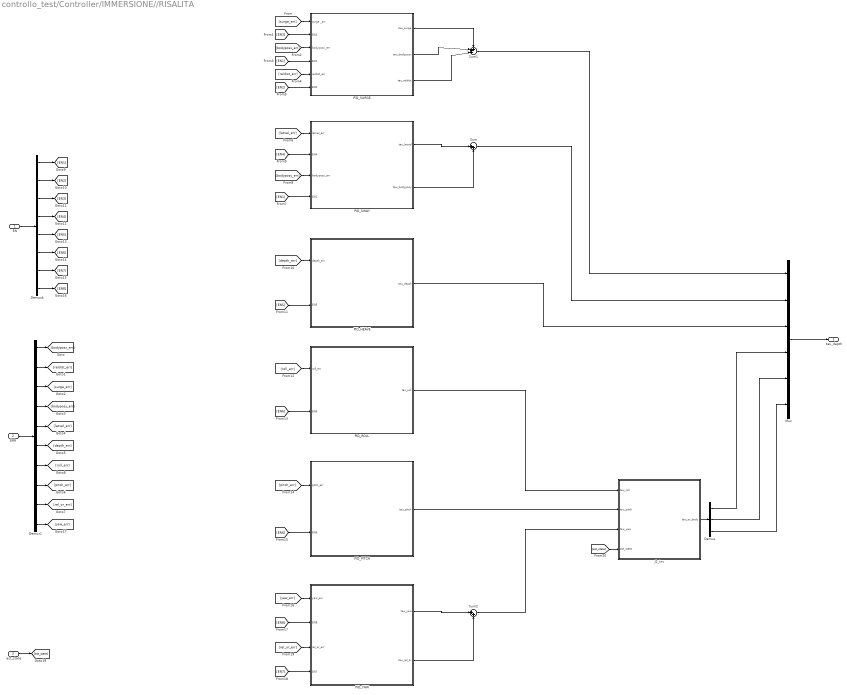
== system controllo_test/Controller/IMMERSIONE//RISALITA ==
  EN : Inport
  ERR : Inport  Port=2
  est_state : Inport  Port=3
  Demux : Demux  Outputs=3
  Demux1 : Demux  Outputs=10
  Demux4 : Demux  Outputs=8
  J2_inv : MATLAB Function  TreatAsAtomicUnit=on
  Mux : Mux  Inputs=6
  PID_HEAVE : Subsystem
  PID_PITCH : Subsystem
  "PID_ROLL " : Subsystem
  PID_SURGE : Subsystem
  PID_SWAY : Subsystem
  PID_YAW : Subsystem
  Sum : Sum  Inputs=|++
  Sum1 : Sum  Inputs=+++|
  Sum2 : Sum  Inputs=|++
  tau_depth : Outport
  wires:
  EN/1 -> Demux4/1
  ERR/1 -> Demux1/1
  Demux4/1 -> [EN1]
  Demux4/2 -> [EN2]
  Demux4/3 -> [EN3]
  Demux4/4 -> [EN4]
  Demux4/5 -> [EN5]
  Demux4/6 -> [EN6]
  Demux4/7 -> [EN7]
  Demux4/8 -> [EN8]
  Demux1/1 -> [bodyposx_err]
  Demux1/2 -> [reldist_err]
  Demux1/3 -> [surge_err]
  Demux1/4 -> [bodyposy_err]
  Demux1/5 -> [latvel_err]
  Demux1/6 -> [depth_err]
  Demux1/7 -> [roll_err]
  Demux1/8 -> [pitch_err]
  Demux1/9 -> [rel_or_err]
  Demux1/10 -> [yaw_err]
  [surge_err] -> PID_SURGE/1(surge _err)
  [EN3] -> PID_SURGE/2(EN3)
  [bodyposx_err] -> PID_SURGE/3(bodyposx_err)
  [EN1] -> PID_SURGE/4(EN1)
  [reldist_err] -> PID_SURGE/5(reldist_err)
  [EN2] -> PID_SURGE/6(EN2)
  [latvel_err] -> PID_SWAY/1(latvel_err)
  [bodyposy_err] -> PID_SWAY/3(bodyposy_err)
  [depth_err] -> PID_HEAVE/1(depth_err)
  [roll_err] -> "PID_ROLL "/1(roll_err)
  [pitch_err] -> PID_PITCH/1(pitch_err)
  [EN6] -> PID_PITCH/2(EN6)
  [yaw_err] -> PID_YAW/1(yaw_err)
  [EN4] -> PID_SWAY/2(EN4)
  [EN1] -> PID_SWAY/4(EN1)
  [EN5] -> PID_HEAVE/2(EN5)
  [EN6] -> "PID_ROLL "/2(EN6)
  [EN8] -> PID_YAW/2("EN8 ")
  [EN7] -> PID_YAW/4(EN7)
  [rel_or_err] -> PID_YAW/3(rel_or_err)
  PID_HEAVE/1(tau_depth) -> Mux/3
  PID_SURGE/1(tau_surge) -> Sum1/1
  Mux/1 -> tau_depth/1
  Sum1/1 -> Mux/1
  Sum/1 -> Mux/2
  PID_YAW/1(tau_yaw) -> Sum2/1
  PID_SWAY/2(tau_bodyposy) -> Sum/2
  PID_SURGE/3(tau_reldist) -> Sum1/3
  PID_SURGE/2(tau_bodyposx) -> Sum1/2
  PID_YAW/2(tau_rel_or) -> Sum2/2
  PID_SWAY/1(tau_latvel) -> Sum/1
  Demux/2 -> Mux/5
  [est_state] -> J2_inv/4(est_state)
  "PID_ROLL "/1(tau_roll) -> J2_inv/1(tau_roll)
  Demux/3 -> Mux/6
  Demux/1 -> Mux/4
  PID_PITCH/1(tau_pitch) -> J2_inv/2(tau_pitch)
  Sum2/1 -> J2_inv/3(tau_yaw)
  J2_inv/1(tau_or_body) -> Demux/1
  est_state/1 -> [est_state]

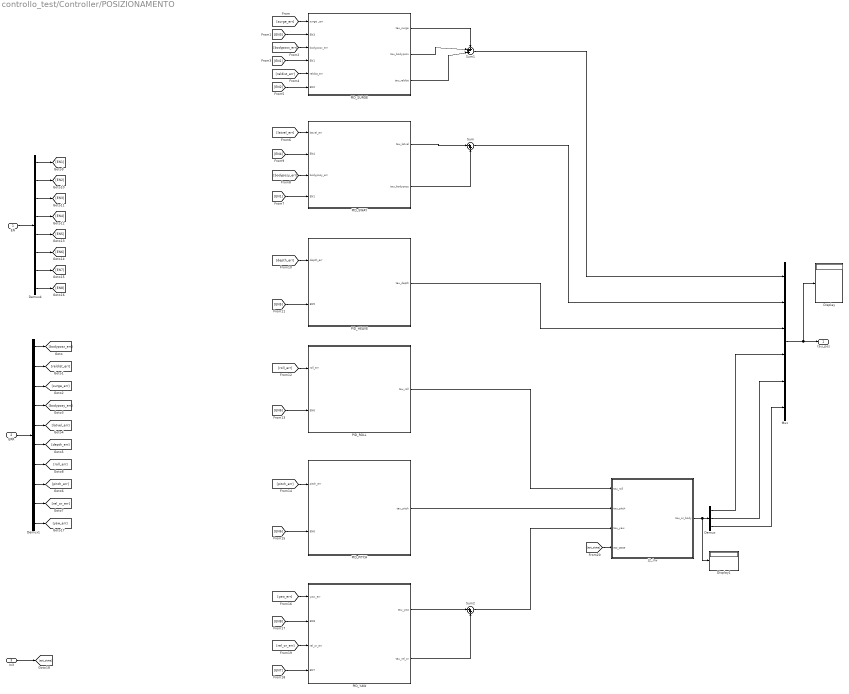
== system controllo_test/Controller/POSIZIONAMENTO ==
  EN : Inport
  ERR : Inport  Port=2
  In3 : Inport  Port=3
  Demux : Demux  Outputs=3
  Demux1 : Demux  Outputs=10
  Demux4 : Demux  Outputs=8
  Display : Display
  Display1 : Display
  J2_inv : MATLAB Function  TreatAsAtomicUnit=on
  Mux : Mux  Inputs=6
  PID_HEAVE : Subsystem
  PID_PITCH : Subsystem
  "PID_ROLL " : Subsystem
  PID_SURGE : Subsystem
  PID_SWAY : Subsystem
  PID_YAW : Subsystem
  Sum : Sum  Inputs=|++
  Sum1 : Sum  Inputs=+++|
  Sum2 : Sum  Inputs=|++
  tau_pos : Outport
  wires:
  PID_SWAY/1(tau_latvel) -> Sum/1
  PID_YAW/2(tau_rel_or) -> Sum2/2
  PID_SURGE/2(tau_bodyposx) -> Sum1/2
  PID_SURGE/3(tau_reldist) -> Sum1/3
  PID_SWAY/2(tau_bodyposy) -> Sum/2
  PID_YAW/1(tau_yaw) -> Sum2/1
  Sum/1 -> Mux/2
  Sum1/1 -> Mux/1
  Mux/1 -> Display/1, tau_pos/1
  PID_SURGE/1(tau_surge) -> Sum1/1
  PID_HEAVE/1(tau_depth) -> Mux/3
  [rel_or_err] -> PID_YAW/3(rel_or_err)
  [EN7] -> PID_YAW/4(EN7)
  [EN8] -> PID_YAW/2("EN8 ")
  [EN6] -> "PID_ROLL "/2(EN6)
  [EN5] -> PID_HEAVE/2(EN5)
  [EN1] -> PID_SWAY/4(EN1)
  [EN4] -> PID_SWAY/2(EN4)
  [yaw_err] -> PID_YAW/1(yaw_err)
  [EN6] -> PID_PITCH/2(EN6)
  [pitch_err] -> PID_PITCH/1(pitch_err)
  [roll_err] -> "PID_ROLL "/1(roll_err)
  [depth_err] -> PID_HEAVE/1(depth_err)
  [bodyposy_err] -> PID_SWAY/3(bodyposy_err)
  [latvel_err] -> PID_SWAY/1(latvel_err)
  [EN2] -> PID_SURGE/6(EN2)
  [reldist_err] -> PID_SURGE/5(reldist_err)
  [EN1] -> PID_SURGE/4(EN1)
  [bodyposx_err] -> PID_SURGE/3(bodyposx_err)
  [EN3] -> PID_SURGE/2(EN3)
  [surge_err] -> PID_SURGE/1(surge _err)
  Demux1/10 -> [yaw_err]
  Demux1/9 -> [rel_or_err]
  Demux1/8 -> [pitch_err]
  Demux1/7 -> [roll_err]
  Demux1/6 -> [depth_err]
  Demux1/5 -> [latvel_err]
  Demux1/4 -> [bodyposy_err]
  Demux1/3 -> [surge_err]
  Demux1/2 -> [reldist_err]
  Demux1/1 -> [bodyposx_err]
  Demux4/8 -> [EN8]
  Demux4/7 -> [EN7]
  Demux4/6 -> [EN6]
  Demux4/5 -> [EN5]
  Demux4/4 -> [EN4]
  Demux4/3 -> [EN3]
  Demux4/2 -> [EN2]
  Demux4/1 -> [EN1]
  ERR/1 -> Demux1/1
  EN/1 -> Demux4/1
  In3/1 -> [est_state]
  [est_state] -> J2_inv/4(est_state)
  "PID_ROLL "/1(tau_roll) -> J2_inv/1(tau_roll)
  PID_PITCH/1(tau_pitch) -> J2_inv/2(tau_pitch)
  Sum2/1 -> J2_inv/3(tau_yaw)
  J2_inv/1(tau_or_body) -> Display1/1, Demux/1
  Demux/1 -> Mux/4
  Demux/2 -> Mux/5
  Demux/3 -> Mux/6

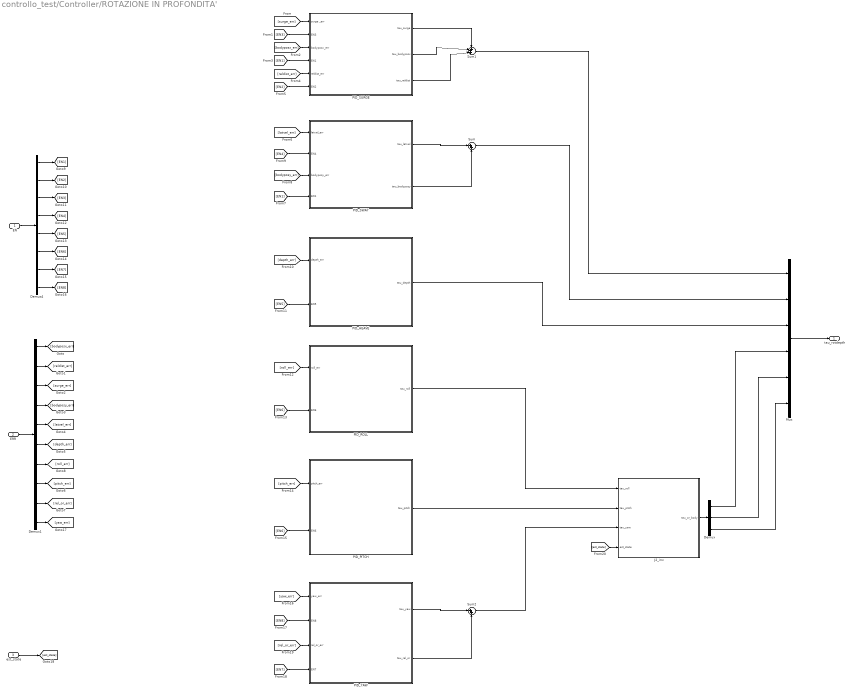
== system controllo_test/Controller/ROTAZIONE IN PROFONDITA' ==
  EN : Inport
  ERR : Inport  Port=2
  est_state : Inport  Port=3
  Demux : Demux  Outputs=3
  Demux1 : Demux  Outputs=10
  Demux4 : Demux  Outputs=8
  J2_inv : MATLAB Function  TreatAsAtomicUnit=on
  Mux : Mux  Inputs=6
  PID_HEAVE : Subsystem
  PID_PITCH : Subsystem
  "PID_ROLL " : Subsystem
  PID_SURGE : Subsystem
  PID_SWAY : Subsystem
  PID_YAW : Subsystem
  Sum : Sum  Inputs=|++
  Sum1 : Sum  Inputs=+++|
  Sum2 : Sum  Inputs=|++
  tau_rotdepth : Outport
  wires:
  EN/1 -> Demux4/1
  ERR/1 -> Demux1/1
  Demux4/1 -> [EN1]
  Demux4/2 -> [EN2]
  Demux4/3 -> [EN3]
  Demux4/4 -> [EN4]
  Demux4/5 -> [EN5]
  Demux4/6 -> [EN6]
  Demux4/7 -> [EN7]
  Demux4/8 -> [EN8]
  Demux1/1 -> [bodyposx_err]
  Demux1/2 -> [reldist_err]
  Demux1/3 -> [surge_err]
  Demux1/4 -> [bodyposy_err]
  Demux1/5 -> [latvel_err]
  Demux1/6 -> [depth_err]
  Demux1/7 -> [roll_err]
  Demux1/8 -> [pitch_err]
  Demux1/9 -> [rel_or_err]
  Demux1/10 -> [yaw_err]
  [surge_err] -> PID_SURGE/1(surge _err)
  [EN3] -> PID_SURGE/2(EN3)
  [bodyposx_err] -> PID_SURGE/3(bodyposx_err)
  [EN1] -> PID_SURGE/4(EN1)
  [reldist_err] -> PID_SURGE/5(reldist_err)
  [EN2] -> PID_SURGE/6(EN2)
  [latvel_err] -> PID_SWAY/1(latvel_err)
  [bodyposy_err] -> PID_SWAY/3(bodyposy_err)
  [depth_err] -> PID_HEAVE/1(depth_err)
  [roll_err] -> "PID_ROLL "/1(roll_err)
  [pitch_err] -> PID_PITCH/1(pitch_err)
  [EN6] -> PID_PITCH/2(EN6)
  [yaw_err] -> PID_YAW/1(yaw_err)
  [EN4] -> PID_SWAY/2(EN4)
  [EN1] -> PID_SWAY/4(EN1)
  [EN5] -> PID_HEAVE/2(EN5)
  [EN6] -> "PID_ROLL "/2(EN6)
  [EN8] -> PID_YAW/2("EN8 ")
  [EN7] -> PID_YAW/4(EN7)
  [rel_or_err] -> PID_YAW/3(rel_or_err)
  PID_HEAVE/1(tau_depth) -> Mux/3
  PID_SURGE/1(tau_surge) -> Sum1/1
  Mux/1 -> tau_rotdepth/1
  Sum1/1 -> Mux/1
  Sum/1 -> Mux/2
  PID_YAW/1(tau_yaw) -> Sum2/1
  PID_SWAY/2(tau_bodyposy) -> Sum/2
  PID_SURGE/3(tau_reldist) -> Sum1/3
  PID_SURGE/2(tau_bodyposx) -> Sum1/2
  PID_YAW/2(tau_rel_or) -> Sum2/2
  PID_SWAY/1(tau_latvel) -> Sum/1
  Demux/1 -> Mux/4
  Sum2/1 -> J2_inv/3(tau_yaw)
  Demux/3 -> Mux/6
  "PID_ROLL "/1(tau_roll) -> J2_inv/1(tau_roll)
  Demux/2 -> Mux/5
  [est_state] -> J2_inv/4(est_state)
  PID_PITCH/1(tau_pitch) -> J2_inv/2(tau_pitch)
  J2_inv/1(tau_or_body) -> Demux/1
  est_state/1 -> [est_state]

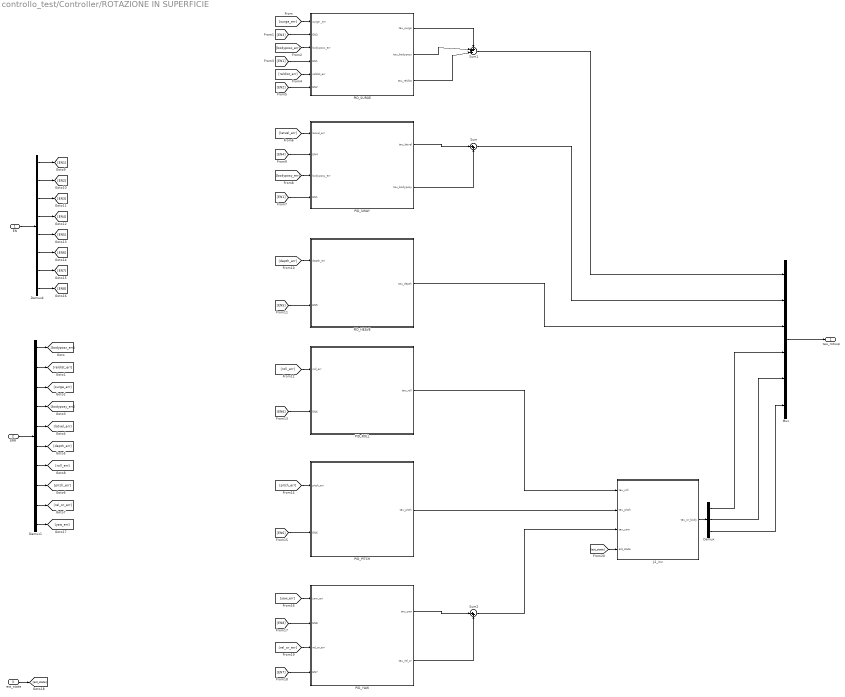
== system controllo_test/Controller/ROTAZIONE IN SUPERFICIE ==
  EN : Inport
  ERR : Inport  Port=2
  est_state : Inport  Port=3
  Demux : Demux  Outputs=3
  Demux1 : Demux  Outputs=10
  Demux4 : Demux  Outputs=8
  J2_inv : MATLAB Function  TreatAsAtomicUnit=on
  Mux : Mux  Inputs=6
  PID_HEAVE : Subsystem
  PID_PITCH : Subsystem
  "PID_ROLL " : Subsystem
  PID_SURGE : Subsystem
  PID_SWAY : Subsystem
  PID_YAW : Subsystem
  Sum : Sum  Inputs=|++
  Sum1 : Sum  Inputs=+++|
  Sum2 : Sum  Inputs=|++
  tau_rotsup : Outport
  wires:
  EN/1 -> Demux4/1
  ERR/1 -> Demux1/1
  Demux4/1 -> [EN1]
  Demux4/2 -> [EN2]
  Demux4/3 -> [EN3]
  Demux4/4 -> [EN4]
  Demux4/5 -> [EN5]
  Demux4/6 -> [EN6]
  Demux4/7 -> [EN7]
  Demux4/8 -> [EN8]
  Demux1/1 -> [bodyposx_err]
  Demux1/2 -> [reldist_err]
  Demux1/3 -> [surge_err]
  Demux1/4 -> [bodyposy_err]
  Demux1/5 -> [latvel_err]
  Demux1/6 -> [depth_err]
  Demux1/7 -> [roll_err]
  Demux1/8 -> [pitch_err]
  Demux1/9 -> [rel_or_err]
  Demux1/10 -> [yaw_err]
  [surge_err] -> PID_SURGE/1(surge _err)
  [EN3] -> PID_SURGE/2(EN3)
  [bodyposx_err] -> PID_SURGE/3(bodyposx_err)
  [EN1] -> PID_SURGE/4(EN1)
  [reldist_err] -> PID_SURGE/5(reldist_err)
  [EN2] -> PID_SURGE/6(EN2)
  [latvel_err] -> PID_SWAY/1(latvel_err)
  [bodyposy_err] -> PID_SWAY/3(bodyposy_err)
  [depth_err] -> PID_HEAVE/1(depth_err)
  [roll_err] -> "PID_ROLL "/1(roll_err)
  [pitch_err] -> PID_PITCH/1(pitch_err)
  [EN6] -> PID_PITCH/2(EN6)
  [yaw_err] -> PID_YAW/1(yaw_err)
  [EN4] -> PID_SWAY/2(EN4)
  [EN1] -> PID_SWAY/4(EN1)
  [EN5] -> PID_HEAVE/2(EN5)
  [EN6] -> "PID_ROLL "/2(EN6)
  [EN8] -> PID_YAW/2("EN8 ")
  [EN7] -> PID_YAW/4(EN7)
  [rel_or_err] -> PID_YAW/3(rel_or_err)
  PID_HEAVE/1(tau_depth) -> Mux/3
  PID_SURGE/1(tau_surge) -> Sum1/1
  Mux/1 -> tau_rotsup/1
  Sum1/1 -> Mux/1
  Sum/1 -> Mux/2
  PID_YAW/1(tau_yaw) -> Sum2/1
  PID_SWAY/2(tau_bodyposy) -> Sum/2
  PID_SURGE/3(tau_reldist) -> Sum1/3
  PID_SURGE/2(tau_bodyposx) -> Sum1/2
  PID_YAW/2(tau_rel_or) -> Sum2/2
  PID_SWAY/1(tau_latvel) -> Sum/1
  J2_inv/1(tau_or_body) -> Demux/1
  "PID_ROLL "/1(tau_roll) -> J2_inv/1(tau_roll)
  Demux/3 -> Mux/6
  Demux/1 -> Mux/4
  PID_PITCH/1(tau_pitch) -> J2_inv/2(tau_pitch)
  [est_state] -> J2_inv/4(est_state)
  Demux/2 -> Mux/5
  Sum2/1 -> J2_inv/3(tau_yaw)
  est_state/1 -> [est_state]

== system controllo_test/Controller/SATURATION ==
  In2 : Inport
  Saturation3 : Saturate  UpperLimit=45  LowerLimit=-45
  Out2 : Outport
  wires:
  In2/1 -> Saturation3/1
  Saturation3/1 -> Out2/1

== system controllo_test/Controller/T2n ==
  Tdes : Inport
  MATLAB Function : MATLAB Function  TreatAsAtomicUnit=on
  n : Outport  Unit=rad/s  PortDimensions=7
  wires:
  Tdes/1 -> MATLAB Function/1(Tdes)
  MATLAB Function/1(n) -> n/1

== system controllo_test/Controller/Tau2T ==
  tau_pos : Inport
  tau_avv : Inport  Port=2
  tau_rotsup : Inport  Port=3
  tau_depth : Inport  Port=4
  tau_rotdepth : Inport  Port=5
  In6 : Inport  Port=6
  Constant : Constant  Value=102
  Data Store Read : DataStoreRead  DataStoreName=current_state  SampleTime=0.1
  Display : Display
  Display1 : Display
  Manual Switch : ManualSwitch
  Tau2T : MATLAB Function  TreatAsAtomicUnit=on
  Tau_des ENABLE : MATLAB Function  TreatAsAtomicUnit=on
  Tdes : Outport
  wires:
  Tau2T/1(T) -> Display1/1, Tdes/1
  tau_avv/1 -> Tau_des ENABLE/3(tau2)
  tau_rotsup/1 -> Tau_des ENABLE/4(tau3)
  tau_depth/1 -> Tau_des ENABLE/5(tau4)
  tau_rotdepth/1 -> Tau_des ENABLE/6(tau5)
  Tau_des ENABLE/1(tau_des) -> Display/1, Tau2T/1(tau_des)
  Constant/1 -> Manual Switch/1
  Manual Switch/1 -> Tau_des ENABLE/1(STATE)
  In6/1 -> Manual Switch/2
  tau_pos/1 -> Tau_des ENABLE/2(tau1)

== system controllo_test/Env. & Sensor Model/AHRS SENSOR ==
  note: AHRS
      |
      | Dynamic Accuracy (Heading):   2.0° RMS
      | Dynamic Accuracy (Pitch/Roll): 1.0° RMS
  note: Output Rate (IMU Data): 800 Hz
  note: Resolution:
  note: 0.02		      	 °
      | 0.3491 * 10-3 rad
  note: 0.05				°
      | 0,8727 * 10^-3	rad
  note: 0,0015 Gauss
  note: Vectornav VN-100 IMU/AHRS
  note: IMU
  note: 0.05			    mg
      | 0.4905 * 10^-3  m/s^2
  note: Output Rate (Attitude Data): 400 Hz
  ni_1 : Inport  SampleTime=IMU_sample_time
  ni_1_dot : Inport  Port=2  SampleTime=IMU_sample_time
  ni_2 : Inport  Port=3  SampleTime=IMU_sample_time
  eta_2 : Inport  Port=4  SampleTime=AHRS_sample_time
  eta_2_dot : Inport  Port=5  SampleTime=IMU_sample_time
  "   " : MATLAB Function  TreatAsAtomicUnit=on
  ACC : Constant
  AHRS2 : Constant
  Accelerometer : Subsystem
  Bus Creator : BusCreator  Inputs=3
  GYRO : Constant
  Gyroscope : Subsystem
  Magnetometer : Subsystem
  Quantizer : Quantizer  QuantizationInterval=Resolution_acc
  Quantizer1 : Quantizer  QuantizationInterval=Resolution_gyro
  Quantizer2 : Quantizer  QuantizationInterval=Resolution_magn
  Quantizer3 : Quantizer  QuantizationInterval=Resolution_AHRS
  Random Number : RandomNumber  Mean=AHRS_bias  Variance=AHRS_var  Seed=[232 342 202]  SampleTime=AHRS_sample_time
  Scope : Scope
  Sum : Sum  Inputs=|++
  Output8 : Outport  SampleTime=IMU_sample_time
  Output9 : Outport  Port=2  SampleTime=IMU_sample_time
  Output10 : Outport  Port=3  SampleTime=AHRS_sample_time
  Output : Outport  Port=4  SampleTime=AHRS_sample_time
  wires:
  "   "/2(ang_vel) -> Gyroscope/1(In1)
  Gyroscope/1(ang_vel) -> Quantizer1/1
  ni_1/1 -> "   "/1(ni_1)
  eta_2/1 -> Sum/2, "   "/4(eta_2)
  ni_2/1 -> "   "/3(ni_2)
  Quantizer2/1 -> Scope/1
  Quantizer1/1 -> Output9/1
  Accelerometer/1(lin_acc) -> Quantizer/1
  ni_1_dot/1 -> "   "/2(ni_1_dot)
  Sum/1 -> Quantizer3/1
  "   "/1(lin_acc) -> Accelerometer/1(In1)
  Quantizer/1 -> Output8/1
  eta_2_dot/1 -> "   "/5(eta_2_dot)
  Random Number/1 -> Sum/1
  "   "/3(m) -> Magnetometer/1(In1)
  Magnetometer/1(m) -> Quantizer2/1
  Quantizer3/1 -> Output10/1
  ACC/1 -> Bus Creator/1
  GYRO/1 -> Bus Creator/2
  AHRS2/1 -> Bus Creator/3
  Bus Creator/1 -> Output/1

== system controllo_test/Env. & Sensor Model/DVL SENSOR ==
  By model2 : Inport  SampleTime=DVL_sample_t
  AND1 : Logic  IconShape=distinctive  AllPortsSameDT=off  OutDataTypeStr=boolean
  DVL : Constant
  Data Type Conversion : DataTypeConversion  OutDataTypeStr=double
  Demux : Demux  Outputs=3
  MATLAB Function : MATLAB Function  TreatAsAtomicUnit=on
  MATLAB Function2 : MATLAB Function  TreatAsAtomicUnit=on
  Quantizer : Quantizer  QuantizationInterval=DVL_resol
  Selector9 : Selector  InputPortWidth=6  IndexOptions=Index vector (dialog)  Indices=[1 2 3]  OutputSizes=1
  Subsystem : Subsystem
  Subsystem1 : Subsystem
  Subsystem2 : Subsystem
  Sum1 : Sum  Inputs=|++
  Sum2 : Sum  Inputs=|++
  Sum3 : Sum  Inputs=|++
  Vector Concatenate : Concatenate  NumInputs=3
  v_sens1 : Outport  SampleTime=DVL_sample_t
  flag_DVL : Outport  Port=2  SampleTime=DVL_sample_t
  wires:
  MATLAB Function2/1(flag) -> AND1/1
  DVL/1 -> AND1/2
  AND1/1 -> Data Type Conversion/1
  Demux/1 -> Sum1/1, Subsystem/1(In1)
  Subsystem/1(Out1) -> Sum1/2
  Demux/2 -> Sum2/1, Subsystem1/1(In1)
  Subsystem1/1(Out1) -> Sum2/2
  Demux/3 -> Sum3/1, Subsystem2/1(In1)
  Subsystem2/1(Out1) -> Sum3/2
  Sum2/1 -> Vector Concatenate/2
  Sum1/1 -> Vector Concatenate/1
  Sum3/1 -> Vector Concatenate/3
  Vector Concatenate/1 -> Quantizer/1
  By model2/1 -> MATLAB Function/1(ni), Selector9/1
  Quantizer/1 -> v_sens1/1
  Data Type Conversion/1 -> flag_DVL/1
  Selector9/1 -> MATLAB Function2/1(v)
  MATLAB Function/1(niDVL) -> Demux/1

== system controllo_test/Env. & Sensor Model/GPS SENSOR ==
  note: Copernicus II DIP
  note: Control state sensors. 1:enabled, 0:disabled
  "[x, y, z] [m]" : Inport  SampleTime=gps_sample_t
  Add noiose : Subsystem
  Control state : Subsystem
  Demux : Demux  Outputs=3
  NED2Geodetic : MATLAB Function  TreatAsAtomicUnit=on
  Threshold : MATLAB Function  TreatAsAtomicUnit=on
  Zero-Order Hold : ZeroOrderHold  SampleTime=gps_sample_t
  Lat e Lon Measure [deg] : Outport
  Flag enable gps : Outport  Port=2
  wires:
  Threshold/2(x_out) -> Add noiose/1(In1)  "x"
  Threshold/3(y_out) -> Add noiose/2(In2)  "y"
  Threshold/1(depth) -> NED2Geodetic/1(depth)
  Add noiose/1(Out1) -> NED2Geodetic/2(u)  "out"
  Threshold/4(flag_enable_gps) -> Control state/1(In1)
  Control state/1(Flag enable gps) -> NED2Geodetic/3(enableGps), Flag enable gps/1
  NED2Geodetic/1(data_GDT) -> Zero-Order Hold/1
  "[x, y, z] [m]"/1 -> Demux/1
  Demux/1 -> Threshold/1(x_in)
  Demux/2 -> Threshold/2(y_in)
  Demux/3 -> Threshold/3(h_in)
  Zero-Order Hold/1 -> Lat e Lon Measure [deg]/1  "(deg/deg/bool)"

== system controllo_test/Env. & Sensor Model/Pressure sensor ==
  h : Inport  SampleTime=ps_sample_t
  orient : Inport  Port=2
  DEPTH MEASUREMENT : Constant
  MATLAB Function2 : MATLAB Function  TreatAsAtomicUnit=on
  MATLAB Function3 : MATLAB Function  TreatAsAtomicUnit=on
  Quantizer1 : Quantizer  QuantizationInterval=ps_resol  LinearizeAsGain=off
  Random Number1 : RandomNumber  Variance=ps_var  SampleTime=ps_sample_t
  Sum1 : Sum  Inputs=|++
  Zero-Order Hold : ZeroOrderHold  SampleTime=ps_sample_t
  Output1 : Outport  SampleTime=ps_sample_t
  Output7 : Outport  Port=2
  wires:
  DEPTH MEASUREMENT/1 -> Output7/1
  Random Number1/1 -> Sum1/2
  MATLAB Function2/1(p) -> Sum1/1
  MATLAB Function3/1(h) -> Zero-Order Hold/1
  Sum1/1 -> Quantizer1/1
  Quantizer1/1 -> MATLAB Function3/2(p)
  h/1 -> MATLAB Function2/1(h)
  Zero-Order Hold/1 -> Output1/1
  orient/1 -> MATLAB Function3/1(orient)

== system controllo_test/Env. & Sensor Model/Sonar sensor ==
  Position (m) (NED) : Inport  SampleTime=s_data.smpl
  Orientation (rad) : Inport  Port=2  SampleTime=s_data.smpl
  Demux : Demux  Outputs=3
  Demux1 : Demux  Outputs=3
  Gain : Gain  Gain=8*ones(5,1)  Multiplication=Matrix(K*u)
  MATLAB Function : MATLAB Function  TreatAsAtomicUnit=on
  MATLAB Function1 : MATLAB Function  TreatAsAtomicUnit=on
  Noises : Subsystem
  Quantizer : Quantizer  QuantizationInterval=s_data.res
  SONAR : Constant  Value=0
  Sum : Sum  Inputs=++|
  Sonar : Outport
  Flag : Outport  Port=2
  wires:
  MATLAB Function/1(s) -> MATLAB Function1/1(s_in)
  MATLAB Function1/1(s_out) -> Sum/2
  Noises/1(Noises) -> Sum/1
  Position (m) (NED)/1 -> Demux/1
  Demux/1 -> MATLAB Function/1(xNorth)
  Demux/2 -> MATLAB Function/2(yEast)
  Demux/3 -> MATLAB Function1/2(depth), MATLAB Function/3(zDown)
  Demux1/3 -> MATLAB Function/6(yaw)
  Demux1/2 -> MATLAB Function/5(pitch)
  Demux1/1 -> MATLAB Function/4(roll)
  Orientation (rad)/1 -> Demux1/1
  SONAR/1 -> Gain/1
  Gain/1 -> MATLAB Function1/3(error)
  Quantizer/1 -> Sonar/1
  MATLAB Function1/2(flag) -> Flag/1
  Sum/1 -> Quantizer/1

== system controllo_test/Navigation1/Geodetic to NED ==
  GPS : Inport
  Depth : Inport  Port=2
  Demux : Demux  Outputs=2
  Demux1 : Demux  Outputs=[2 1]
  Gain1 : Gain  Gain=pi/180
  MATLAB Function2 : MATLAB Function  TreatAsAtomicUnit=on
  Terminator : Terminator
  GPS_NED : Outport
  wires:
  Demux1/2 -> MATLAB Function2/2(GPS_flag)
  MATLAB Function2/1(GPS_NED) -> GPS_NED/1
  GPS/1 -> Demux1/1
  Demux1/1 -> Gain1/1
  Gain1/1 -> MATLAB Function2/1(GPS_geodetic)
  Depth/1 -> Demux/1
  Demux/1 -> MATLAB Function2/3(depth)
  Demux/2 -> Terminator/1

== system controllo_test/Navigation1/Geodetic to NED1 ==
  GPS : Inport
  Depth : Inport  Port=2
  Demux : Demux  Outputs=2
  Demux1 : Demux  Outputs=[2 1]
  Gain1 : Gain  Gain=pi/180
  MATLAB Function2 : MATLAB Function  TreatAsAtomicUnit=on
  Terminator : Terminator
  GPS_NED : Outport
  wires:
  Demux1/2 -> MATLAB Function2/2(GPS_flag)
  MATLAB Function2/1(GPS_NED) -> GPS_NED/1
  GPS/1 -> Demux1/1
  Demux1/1 -> Gain1/1
  Gain1/1 -> MATLAB Function2/1(GPS_geodetic)
  Depth/1 -> Demux/1
  Demux/1 -> MATLAB Function2/3(depth)
  Demux/2 -> Terminator/1
